simulink model "mixer"  (R2019b)
settings: Solver=VariableStepAuto  StartTime=0.0  StopTime=1000.00  RelTol=1e-3
model workspace (MAT data in the model file):
  V0 = 1
settings Model: Creator=Анастасия  LastModifiedBy=Анастасия

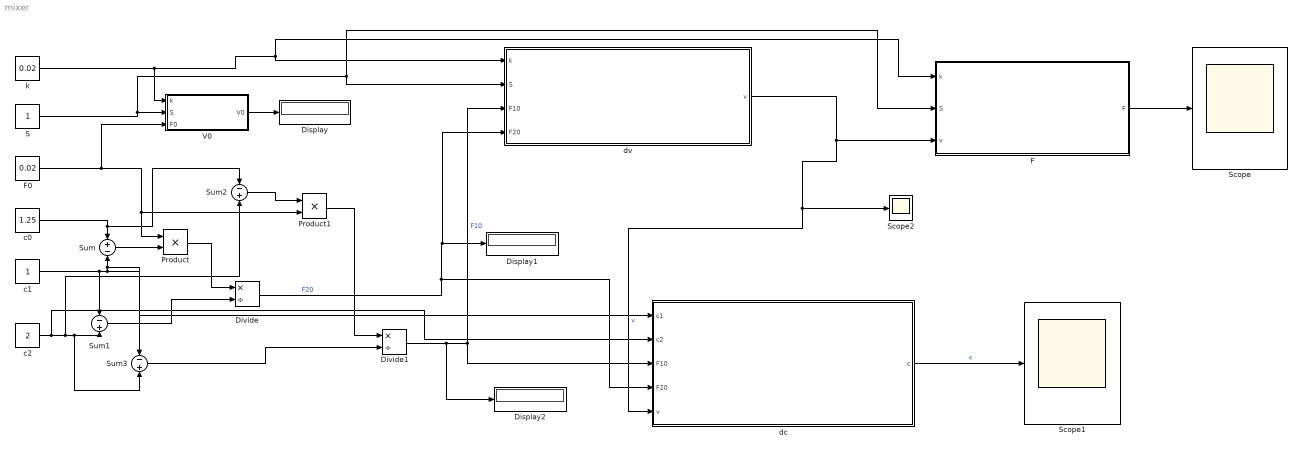
== system mixer ==
  Display : Display
  Display1 : Display
  Display2 : Display
  Divide : Product  Inputs=*/
  Divide1 : Product  Inputs=*/
  F : Subsystem
  F0 : Constant  Value=0.02
  Product : Product
  Product1 : Product
  S : Constant
  Scope : Scope
  Scope1 : Scope
  Scope2 : Scope
  Sum : Sum  Inputs=+-
  Sum1 : Sum  Inputs=-+
  Sum2 : Sum  Inputs=-+
  Sum3 : Sum  Inputs=-+
  V0 : Subsystem
  "c0 " : Constant  Value=1.25
  c1 : Constant
  c2 : Constant  Value=2
  dc : Subsystem
  dv : Subsystem
  k : Constant  Value=0.02
  wires:
  "c0 "/1 -> Sum2/1, Sum/1
  c1/1 -> dc/1(c1), Sum3/1, Sum/2, Sum1/1
  Sum/1 -> Product/2
  F0/1 -> V0/3(F0), Product1/2, Product/1
  c2/1 -> dc/2(c2), Sum2/2, Sum3/2, Sum1/2
  Product/1 -> Divide/1
  Sum1/1 -> Divide/2
  Divide/1 -> dv/4(F20), Display1/1, dc/4(F20)  "F20"
  Sum2/1 -> Product1/1
  Product1/1 -> Divide1/1
  Sum3/1 -> Divide1/2
  Divide1/1 -> Display2/1, dc/3(F10), dv/3(F10)  "F10"
  k/1 -> V0/1(k), F/1(k), dv/1(k)
  S/1 -> V0/2(S), F/2(S), dv/2(S)
  dv/1(v) -> F/3(v), Scope2/1, dc/5(v)  "v"
  dc/1(c) -> Scope1/1  "c"
  F/1(F) -> Scope/1
  V0/1(V0) -> Display/1

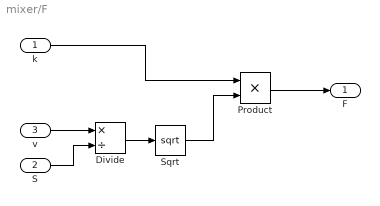
== system mixer/F ==
  k : Inport
  S : Inport  Port=2
  v : Inport  Port=3
  Divide : Product  Inputs=*/
  Product : Product
  Sqrt : Sqrt  SaturateOnIntegerOverflow=on
  F : Outport
  wires:
  k/1 -> Product/1
  S/1 -> Divide/2
  Divide/1 -> Sqrt/1
  Sqrt/1 -> Product/2
  v/1 -> Divide/1
  Product/1 -> F/1

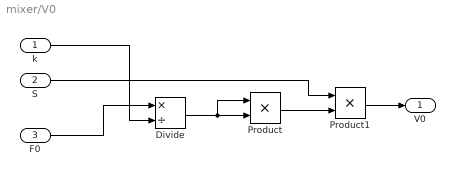
== system mixer/V0 ==
  k : Inport
  S : Inport  Port=2
  F0 : Inport  Port=3
  Divide : Product  Inputs=*/
  Product : Product
  Product1 : Product
  V0 : Outport
  wires:
  F0/1 -> Divide/1
  k/1 -> Divide/2
  Divide/1 -> Product/1, Product/2
  Product/1 -> Product1/2
  S/1 -> Product1/1
  Product1/1 -> V0/1

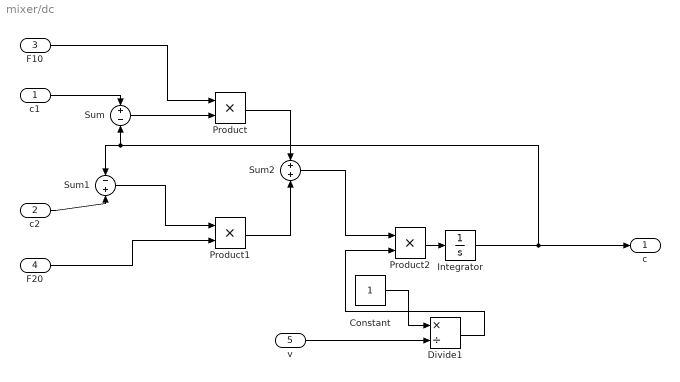
== system mixer/dc ==
  c1 : Inport
  c2 : Inport  Port=2
  F10 : Inport  Port=3
  F20 : Inport  Port=4
  v : Inport  Port=5
  Constant : Constant
  Divide1 : Product  Inputs=*/
  Integrator : Integrator
  Product : Product
  Product1 : Product
  Product2 : Product
  Sum : Sum  Inputs=+-
  Sum1 : Sum  Inputs=-+
  Sum2 : Sum
  c : Outport
  wires:
  c1/1 -> Sum/1
  Integrator/1 -> Sum1/1, Sum/2, c/1
  c2/1 -> Sum1/2
  Sum/1 -> Product/2
  F10/1 -> Product/1
  Sum1/1 -> Product1/1
  F20/1 -> Product1/2
  Product/1 -> Sum2/1
  Product1/1 -> Sum2/2
  Sum2/1 -> Product2/1
  v/1 -> Divide1/2
  Product2/1 -> Integrator/1
  Constant/1 -> Divide1/1
  Divide1/1 -> Product2/2

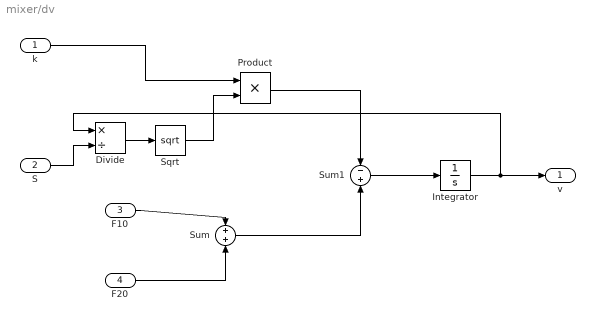
== system mixer/dv ==
  k : Inport
  S : Inport  Port=2
  F10 : Inport  Port=3
  F20 : Inport  Port=4
  Divide : Product  Inputs=*/
  Integrator : Integrator  InitialCondition=1.25
  Product : Product
  Sqrt : Sqrt  SaturateOnIntegerOverflow=on
  Sum : Sum
  Sum1 : Sum  Inputs=-+
  v : Outport
  wires:
  S/1 -> Divide/2
  Divide/1 -> Sqrt/1
  Sqrt/1 -> Product/2
  k/1 -> Product/1
  F10/1 -> Sum/1
  F20/1 -> Sum/2
  Product/1 -> Sum1/1
  Sum/1 -> Sum1/2
  Sum1/1 -> Integrator/1
  Integrator/1 -> Divide/1, v/1
